simulink model "OneIRsensor"  (R2019a)
settings: Solver=FixedStepAuto  StartTime=0.0  StopTime=10.0  RelTol=1e-3
libraries: vexarmcortexlib x21, vexcommonlib x3
settings Model: ExtModeTrigDuration=25  Creator=hsstudent  LastModifiedBy=hsstudent
settings SolverCC: AutoInsertRateTranBlk=on
settings OptimizationCC: EnhancedBackFolding=on  PassReuseOutputArgsAs=Individual arguments  MaxStackSize=64  OptimizeBlockOrder=speed  DifferentSizesBufferReuse=on  OptimizationCustomize=off
settings DebuggingCC: ParameterTunabilityLossMsg=error
settings HardwareCC: ProdBitPerPointer=32  ProdBitPerSizeT=32  ProdBitPerPtrDiffT=32  ProdLargestAtomicInteger=Long  ProdLargestAtomicFloat=Double  ProdWordSize=32  ProdHWDeviceType=ARM Compatible->ARM Cortex
settings SFSimCC: MATLABDynamicMemAlloc=off
settings RTWCC: SystemTargetFile=ert.tlc  HardwareBoard=ARM Cortex-based VEX Microcontroller  TLCOptions="-aInlineSetEventsForThisBaseRateFcn=TLC_FALSE -aSuppressMultiTaskScheduler=TLC_FALSE  -aRateBasedStepFcn=0"  TemplateMakefile=ert_default_tmf  GenerateReport=on  Toolchain=GNU Tools for VEX ARM Cortex  IncludeHyperlinkInReport=on  LaunchReport=on  GenerateTraceInfo=on  GenerateTraceReport=on  GenerateTraceReportSl=on  GenerateTraceReportSf=on  GenerateTraceReportEml=on
settings CodeAppCC: ForceParamTrailComments=on  IgnoreCustomStorageClasses=off  OperatorAnnotations=on  SimulinkDataObjDesc=on  SFDataObjDesc=on  InsertBlockDesc=on

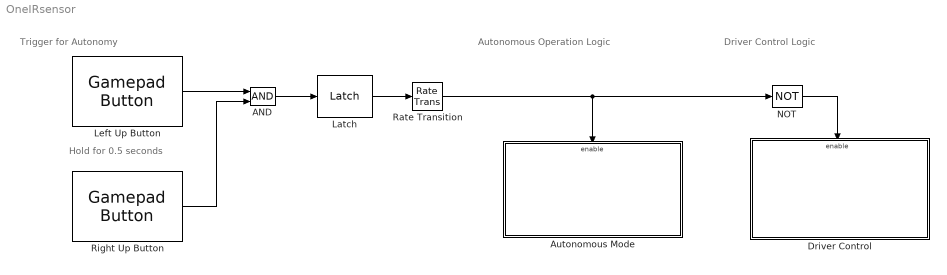
== system OneIRsensor ==
  note: Autonomous Operation Logic
  note: Hold for 0.5 seconds
  note: Driver Control Logic
  note: Trigger for Autonomy
  AND : Logic  IconShape=distinctive  AllPortsSameDT=off  OutDataTypeStr=boolean
  Autonomous Mode : Subsystem
  Driver Control : Subsystem  TreatAsAtomicUnit=on
  Latch : vexcommonlib/Latch  output0=off  BlockPlatform=vexarmcortex
      settings: SourceProductName=Simulink Coder Support Package for ARM Cortex-based VEX Microcontroller  SourceProductBaseCode=EC_VEX_MICRO
  Left Up Button : vexarmcortexlib/Gamepad/Gamepad Button  joystick=1  chan=7  button56=Down  button78=Up  SimulationIn=off  SampleTime=0.5
      settings: SourceProductName=Simulink Coder Support Package for ARM Cortex-based VEX Microcontroller  SourceProductBaseCode=EC_VEX_MICRO
  NOT : Logic  Operator=NOT  IconShape=distinctive  AllPortsSameDT=off  OutDataTypeStr=boolean
  Rate Transition : RateTransition
  Right Up Button : vexarmcortexlib/Gamepad/Gamepad Button  joystick=1  chan=8  button56=Down  button78=Up  SimulationIn=off  SampleTime=0.5
      settings: SourceProductName=Simulink Coder Support Package for ARM Cortex-based VEX Microcontroller  SourceProductBaseCode=EC_VEX_MICRO
  wires:
  Right Up Button/1 -> AND/2
  Left Up Button/1 -> AND/1
  Latch/1 -> Rate Transition/1
  Rate Transition/1 -> NOT/1, Autonomous Mode/Enable
  AND/1 -> Latch/1
  NOT/1 -> Driver Control/Enable

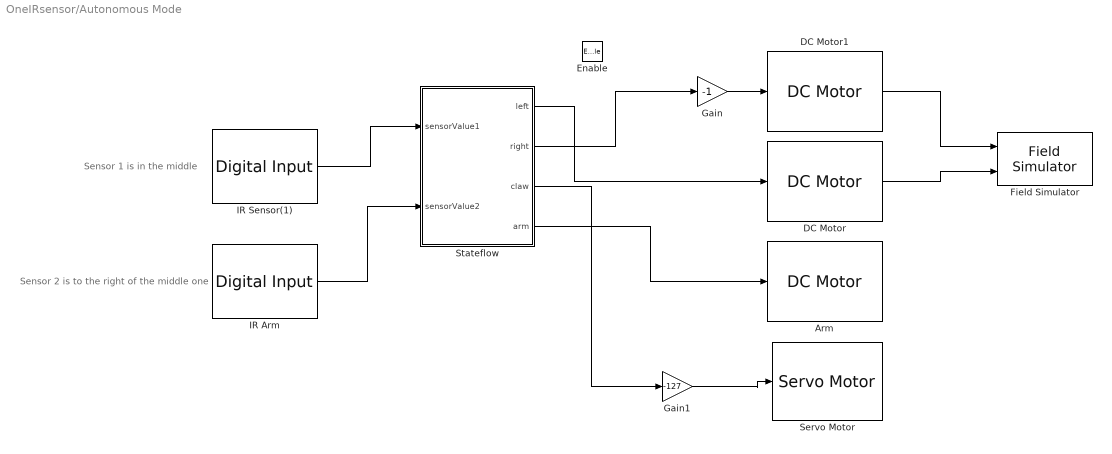
== system OneIRsensor/Autonomous Mode ==
  note: Sensor 2 is to the right of the middle one
  note: Sensor 1 is in the middle
  Enable : EnablePort  StatesWhenEnabling=reset
  Arm : vexarmcortexlib/Actuators/DC Motor  motor=9  scaleFactor=1/13.5  SimulationOut=off
      settings: SourceProductName=Simulink Coder Support Package for ARM Cortex-based VEX Microcontroller  SourceProductBaseCode=EC_VEX_MICRO
  DC Motor : vexarmcortexlib/Actuators/DC Motor  motor=6  scaleFactor=1/13.5  SimulationOut=on
      settings: SourceProductName=Simulink Coder Support Package for ARM Cortex-based VEX Microcontroller  SourceProductBaseCode=EC_VEX_MICRO
  DC Motor1 : vexarmcortexlib/Actuators/DC Motor  motor=2  scaleFactor=1/13.5  SimulationOut=on
      settings: SourceProductName=Simulink Coder Support Package for ARM Cortex-based VEX Microcontroller  SourceProductBaseCode=EC_VEX_MICRO
  Field Simulator : vexcommonlib/Field Simulator  radius=2.5  space=10  range=200  BlockPlatform=vexarmcortex
      settings: SourceProductName=Simulink Coder Support Package for ARM Cortex-based VEX Microcontroller  SourceProductBaseCode=EC_VEX_MICRO
  Gain : Gain  Gain=-1
  Gain1 : Gain  Gain=-127
  "IR Arm " : vexarmcortexlib/Sensors/Digital Input  inChan=4  SimulationIn=off  SampleTime=0.05
      settings: SourceProductName=Simulink Coder Support Package for ARM Cortex-based VEX Microcontroller  SourceProductBaseCode=EC_VEX_MICRO
  IR Sensor(1) : vexarmcortexlib/Sensors/Digital Input  inChan=9  SimulationIn=off  SampleTime=0.05
      settings: SourceProductName=Simulink Coder Support Package for ARM Cortex-based VEX Microcontroller  SourceProductBaseCode=EC_VEX_MICRO
  Servo Motor : vexarmcortexlib/Actuators/Servo Motor  motor=3  scaleFactor=60/127  SimulationOut=off
      settings: SourceProductName=Simulink Coder Support Package for ARM Cortex-based VEX Microcontroller  SourceProductBaseCode=EC_VEX_MICRO
  Stateflow : Stateflow chart  TreatAsAtomicUnit=on
  wires:
  DC Motor/1 -> Field Simulator/2
  Gain/1 -> DC Motor1/1
  DC Motor1/1 -> Field Simulator/1
  Stateflow/1(left) -> DC Motor/1
  Stateflow/2(right) -> Gain/1
  IR Sensor(1)/1 -> Stateflow/1(sensorValue1)
  "IR Arm "/1 -> Stateflow/2(sensorValue2)
  Stateflow/4(arm) -> Arm/1
  Stateflow/3(claw) -> Gain1/1
  Gain1/1 -> Servo Motor/1

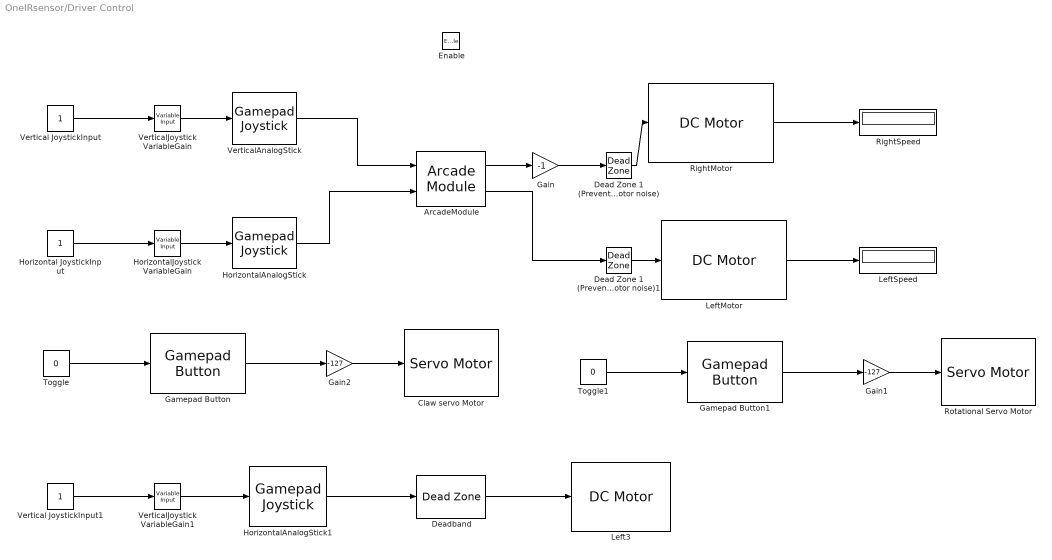
== system OneIRsensor/Driver Control ==
  Enable : EnablePort  StatesWhenEnabling=reset
  ArcadeModule : vexcommonlib/Arcade Module  BlockPlatform=vexarmcortex
      settings: SourceProductName=Simulink Coder Support Package for ARM Cortex-based VEX Microcontroller  SourceProductBaseCode=EC_VEX_MICRO
  Claw servo Motor : vexarmcortexlib/Actuators/Servo Motor  motor=3  scaleFactor=60/127  SimulationOut=on
      settings: SourceProductName=Simulink Coder Support Package for ARM Cortex-based VEX Microcontroller  SourceProductBaseCode=EC_VEX_MICRO
  Dead Zone 1 (Prevents motor noise) : DeadZone  LowerValue=-30  UpperValue=30  SaturateOnIntegerOverflow=on
  Dead Zone 1 (Prevents motor noise)1 : DeadZone  LowerValue=-30  UpperValue=30  SaturateOnIntegerOverflow=on
  Deadband : DeadZone  SaturateOnIntegerOverflow=on
  Gain : Gain  Gain=-1
  Gain1 : Gain  Gain=-127
  Gain2 : Gain  Gain=-127
  Gamepad Button : vexarmcortexlib/Gamepad/Gamepad Button  joystick=1  chan=7  button56=Up  button78=Down  SimulationIn=on  SampleTime=0.02
      settings: SourceProductName=Simulink Coder Support Package for ARM Cortex-based VEX Microcontroller  SourceProductBaseCode=EC_VEX_MICRO
  Gamepad Button1 : vexarmcortexlib/Gamepad/Gamepad Button  joystick=1  chan=8  button56=Up  button78=Down  SimulationIn=on  SampleTime=0.02
      settings: SourceProductName=Simulink Coder Support Package for ARM Cortex-based VEX Microcontroller  SourceProductBaseCode=EC_VEX_MICRO
  Horizontal JoystickInput : Constant
  HorizontalAnalogStick : vexarmcortexlib/Gamepad/Gamepad Joystick  joystick=1  chan=1  SimulationIn=on  SampleTime=0.02
      settings: SourceProductName=Simulink Coder Support Package for ARM Cortex-based VEX Microcontroller  SourceProductBaseCode=EC_VEX_MICRO
  HorizontalAnalogStick1 : vexarmcortexlib/Gamepad/Gamepad Joystick  joystick=1  chan=3  SimulationIn=on  SampleTime=0.02
      settings: SourceProductName=Simulink Coder Support Package for ARM Cortex-based VEX Microcontroller  SourceProductBaseCode=EC_VEX_MICRO
  HorizontalJoystick VariableGain : vexarmcortexlib/Utilities/Variable Input  low=-127  gain=-118.8065  high=127
      settings: SourceProductName=Simulink Coder Support Package for ARM Cortex-based VEX Microcontroller  SourceProductBaseCode=EC_VEX_MICRO
  Left3 : vexarmcortexlib/Actuators/DC Motor  motor=9  scaleFactor=1/13.5  SimulationOut=on
      settings: SourceProductName=Simulink Coder Support Package for ARM Cortex-based VEX Microcontroller  SourceProductBaseCode=EC_VEX_MICRO
  LeftMotor : vexarmcortexlib/Actuators/DC Motor  motor=6  scaleFactor=1/13.5  SimulationOut=on
      settings: SourceProductName=Simulink Coder Support Package for ARM Cortex-based VEX Microcontroller  SourceProductBaseCode=EC_VEX_MICRO
  LeftSpeed : Display
  RightMotor : vexarmcortexlib/Actuators/DC Motor  motor=2  scaleFactor=1/13.5  SimulationOut=on
      settings: SourceProductName=Simulink Coder Support Package for ARM Cortex-based VEX Microcontroller  SourceProductBaseCode=EC_VEX_MICRO
  RightSpeed : Display
  "Rotational Servo Motor " : vexarmcortexlib/Actuators/Servo Motor  motor=8  scaleFactor=60/127  SimulationOut=on
      settings: SourceProductName=Simulink Coder Support Package for ARM Cortex-based VEX Microcontroller  SourceProductBaseCode=EC_VEX_MICRO
  Toggle : Constant  Value=0
      settings: OpenFcn=|
      | if strcmp('0',get_param(gcb, 'Value'))                        set_param(gcb, 'Value', '1');
      | else
      |             set_param(gcb, 'Value', '0');
      | end
  Toggle1 : Constant  Value=0
      settings: OpenFcn=|
      | if strcmp('0',get_param(gcb, 'Value'))                        set_param(gcb, 'Value', '1');
      | else
      |             set_param(gcb, 'Value', '0');
      | end
  Vertical JoystickInput : Constant
  Vertical JoystickInput1 : Constant
  VerticalAnalogStick : vexarmcortexlib/Gamepad/Gamepad Joystick  joystick=1  chan=2  SimulationIn=on  SampleTime=0.02
      settings: SourceProductName=Simulink Coder Support Package for ARM Cortex-based VEX Microcontroller  SourceProductBaseCode=EC_VEX_MICRO
  VerticalJoystick VariableGain : vexarmcortexlib/Utilities/Variable Input  low=-127  gain=0  high=127
      settings: SourceProductName=Simulink Coder Support Package for ARM Cortex-based VEX Microcontroller  SourceProductBaseCode=EC_VEX_MICRO
  VerticalJoystick VariableGain1 : vexarmcortexlib/Utilities/Variable Input  low=-127  gain=-68  high=127
      settings: SourceProductName=Simulink Coder Support Package for ARM Cortex-based VEX Microcontroller  SourceProductBaseCode=EC_VEX_MICRO
  wires:
  Gain2/1 -> Claw servo Motor/1
  Toggle/1 -> Gamepad Button/1
  Dead Zone 1 (Prevents motor noise)/1 -> RightMotor/1
  VerticalJoystick VariableGain1/1 -> HorizontalAnalogStick1/1
  Vertical JoystickInput1/1 -> VerticalJoystick VariableGain1/1
  Dead Zone 1 (Prevents motor noise)1/1 -> LeftMotor/1
  HorizontalAnalogStick1/1 -> Deadband/1
  ArcadeModule/1 -> Gain/1
  Vertical JoystickInput/1 -> VerticalJoystick VariableGain/1
  VerticalJoystick VariableGain/1 -> VerticalAnalogStick/1
  RightMotor/1 -> RightSpeed/1
  HorizontalJoystick VariableGain/1 -> HorizontalAnalogStick/1
  LeftMotor/1 -> LeftSpeed/1
  ArcadeModule/2 -> Dead Zone 1 (Prevents motor noise)1/1
  Horizontal JoystickInput/1 -> HorizontalJoystick VariableGain/1
  Gamepad Button/1 -> Gain2/1
  Gain/1 -> Dead Zone 1 (Prevents motor noise)/1
  VerticalAnalogStick/1 -> ArcadeModule/1
  HorizontalAnalogStick/1 -> ArcadeModule/2
  Deadband/1 -> Left3/1
  Toggle1/1 -> Gamepad Button1/1
  Gain1/1 -> "Rotational Servo Motor "/1
  Gamepad Button1/1 -> Gain1/1

== stateflow chart OneIRsensor/Autonomous Mode/Stateflow ==
  state TowerDetect1
    entry:
    arm = 50;
    left = 0;
    right = 0;
  state Drop
    entry:
    claw = 0;
    arm = 0;
  state GoForward
    entry:
    left = 100;
    right = 100;
  state Stop
    entry:
    left = 0;
    right= 0;
  state Return
    entry:
    arm = -50;
    claw = 0;
  state GoLeft
    entry:
    left = -50
    right = 50
  state Preset
    entry:
    arm = 0;
    claw = 1;
  state Stop2
    entry:
    arm = 0;
    claw = 1;
  state GoRight
    entry:
    left = 50
    right = -50
  state Stop1
    during:
    left = 0
    right = 0
  GoForward -> GoLeft : [sensorValue1 == 1]
  (default) -> Stop [order 1]
  TowerDetect1 -> Drop : after(2,sec)
  Stop -> GoForward : [sensorValue1 == 0]
  Drop -> Return
  GoLeft -> GoForward [order 2] : after(2,sec)[sensorValue1 == 0]
  Preset -> TowerDetect1 : [sensorValue1 == 0, sensorValue2 == 0]
  GoRight -> GoForward [order 2] : [sensorValue1 == 0]
  (default) -> Preset [order 2]
  Return -> Stop2 : after(2,sec)
  GoLeft -> Stop1 [order 1] : after(1.25,sec)[sensorValue1 == 1]
  GoRight -> Stop1 [order 1] : after(2,sec)[sensorValue1 == 1]
  Stop1 -> GoRight : [sensorValue1 == 1]
  data: left output; right output; sensorValue1 input; sensorValue2 input; claw output; arm output
